simulink model "sparse_learning_recalling"  (R2021b)
settings: Solver=VariableStepAuto  StartTime=0.0  StopTime=20.0  RelTol=1e-3
libraries: wnnlib x3
settings Model: Creator=20214358  LastModifiedBy=20214358

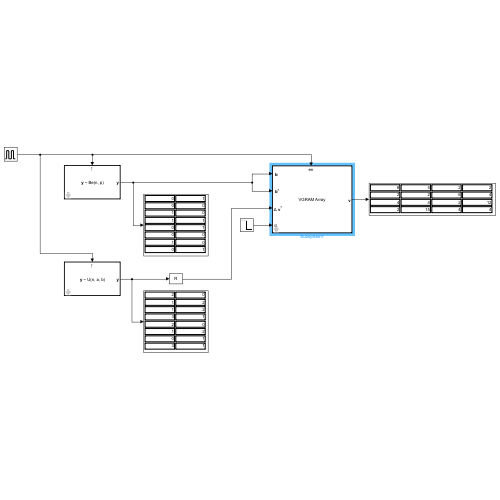
[thumbnail: Simulink's stored preview of the top-level diagram]
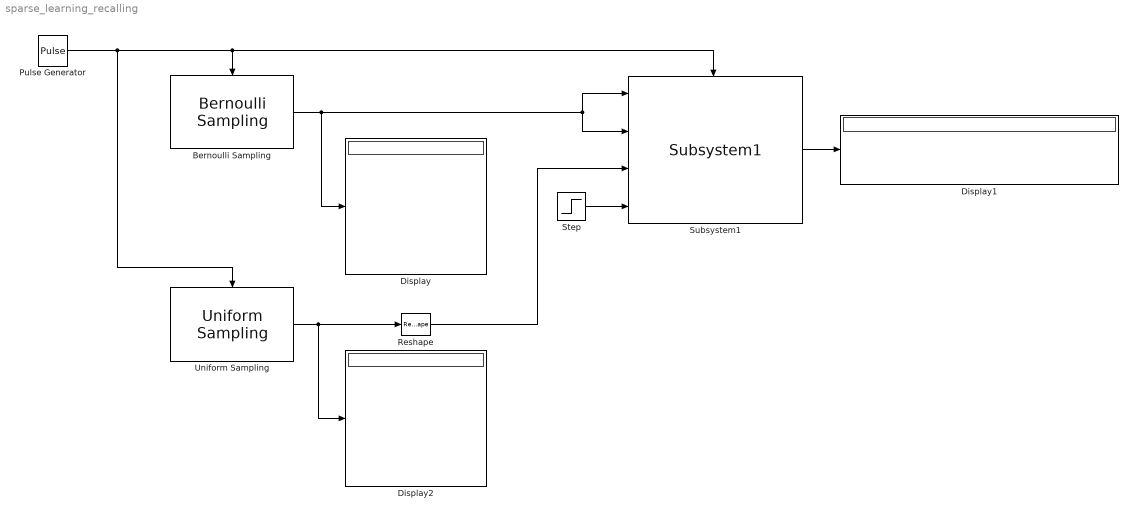
== system sparse_learning_recalling ==
  Bernoulli Sampling : wnnlib/Sources/Bernoulli Sampling  nSamples=16  probability=0.5  nSeed=0
      settings: SourceProductName=Weightless Neural Networks Toolbox
  Display : Display
  Display1 : Display
  Display2 : Display
  Pulse Generator : DiscretePulseGenerator  PulseType=Time based  Period=0.05  PulseWidth=5
  Reshape : Reshape  OutputDimensionality=Customize  OutputDimensions=[4,4]
  Step : Step  Time=10  Before=1  After=0  OutDataTypeStr=Inherit: Inherit via back propagation  SampleTime=0.01
  Subsystem1 : wnnlib/Models/Subsystem1  array_id=0  min_mem_size=63  max_mem_size=64  min_dist=2  max_dist=8  pattern_length=16  output_dims=[4, 4]  debug_flag=on
      settings: SourceProductName=Weightless Neural Networks Toolbox
  Uniform Sampling : wnnlib/Sources/Uniform Sampling  nSamples=16  min_value=0  max_value=3  nSeed=1
      settings: SourceProductName=Weightless Neural Networks Toolbox
  wires:
  Bernoulli Sampling/1 -> Subsystem1/2, Subsystem1/1, Display/1
  Subsystem1/1 -> Display1/1
  Pulse Generator/1 -> Uniform Sampling/Trigger, Subsystem1/Enable, Bernoulli Sampling/Trigger
  Uniform Sampling/1 -> Reshape/1, Display2/1
  Step/1 -> Subsystem1/4
  Reshape/1 -> Subsystem1/3
